simulink model "lab5_model"  (R2024b)
settings: Solver=ode45  StartTime=0.0  StopTime=150  MaxStep=0.05  RelTol=1e-3
libraries: simulink x2
settings Model: Creator=gm54508  LastModifiedBy=gm54508

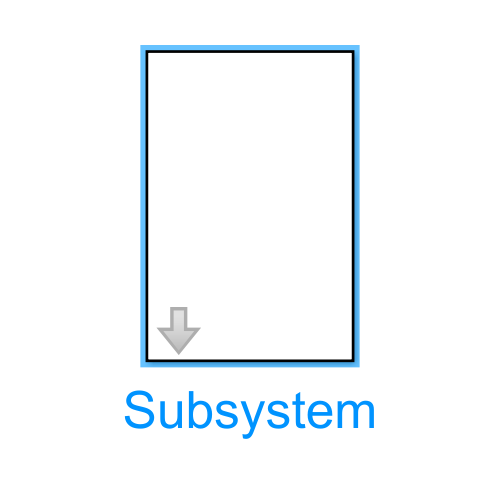
[thumbnail: Simulink's stored preview of the top-level diagram]
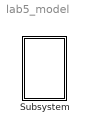
== system lab5_model ==
  Subsystem : Subsystem  mask{h1=6, h2=3, s1=1, s2=2, swy1=0.4, swy2=0.3, fi1=1, fi2=1, g=9.81, qwe=0}

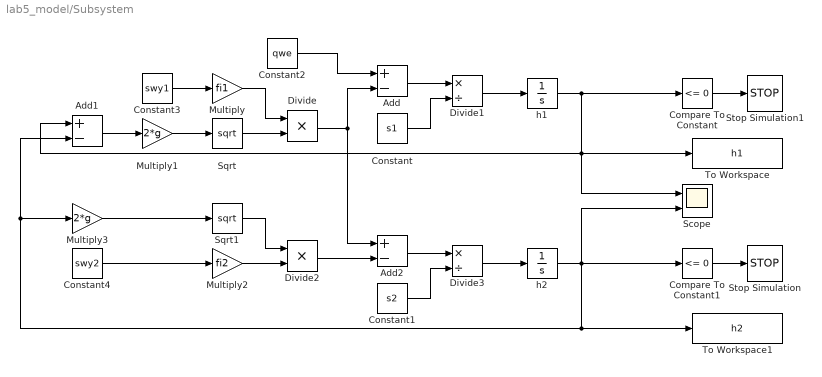
== system lab5_model/Subsystem ==
  Add : Sum  Inputs=+-
  Add1 : Sum  Inputs=+-
  Add2 : Sum  Inputs=+-
  Compare To Constant : simulink/Logic and Bit Operations/Compare To Constant  relop=<=  const=0  OutDataTypeStr=boolean
  Compare To Constant1 : simulink/Logic and Bit Operations/Compare To Constant  relop=<=  const=0  OutDataTypeStr=boolean
  Constant : Constant  Value=s1
  Constant1 : Constant  Value=s2
  Constant2 : Constant  Value=qwe
  Constant3 : Constant  Value=swy1
  Constant4 : Constant  Value=swy2
  Divide : Product  Inputs=**
  Divide1 : Product  Inputs=*/
  Divide2 : Product  Inputs=**
  Divide3 : Product  Inputs=*/
  Multiply : Gain  Gain=fi1
  Multiply1 : Gain  Gain=2*g
  Multiply2 : Gain  Gain=fi2
  Multiply3 : Gain  Gain=2*g
  Scope : Scope  NumInputPorts=2
  Sqrt : Sqrt
  Sqrt1 : Sqrt
  Stop Simulation : Stop
  Stop Simulation1 : Stop
  To Workspace : ToWorkspace  VariableName=h1  SampleTime=-1
  To Workspace1 : ToWorkspace  VariableName=h2  SampleTime=-1
  h1 : Integrator  InitialCondition=h1
  h2 : Integrator  InitialCondition=h2
  wires:
  Add1/1 -> Multiply1/1
  h2/1 -> Scope/2, Compare To Constant1/1, To Workspace1/1, Add1/2, Multiply3/1
  Sqrt/1 -> Divide/2
  h1/1 -> Scope/1, Add1/1, To Workspace/1, Compare To Constant/1
  Divide2/1 -> Add2/2
  Constant4/1 -> Multiply2/1
  Constant3/1 -> Multiply/1
  Divide1/1 -> h1/1
  Multiply1/1 -> Sqrt/1
  Multiply2/1 -> Divide2/2
  Divide3/1 -> h2/1
  Multiply/1 -> Divide/1
  Constant2/1 -> Add/1
  Sqrt1/1 -> Divide2/1
  Compare To Constant1/1 -> Stop Simulation/1
  Divide/1 -> Add2/1, Add/2
  Compare To Constant/1 -> Stop Simulation1/1
  Constant/1 -> Divide1/2
  Constant1/1 -> Divide3/2
  Multiply3/1 -> Sqrt1/1
  Add/1 -> Divide1/1
  Add2/1 -> Divide3/1
